simulink library "utils"  (R2007a)
settings: Solver=ode45  StartTime=0.0  StopTime=10.0  RelTol=1e-3
settings Model: Creator=aeagr  LastModifiedBy=aeagr

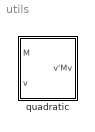
== system utils ==
  quadratic : Subsystem  mask(Quadratic){}

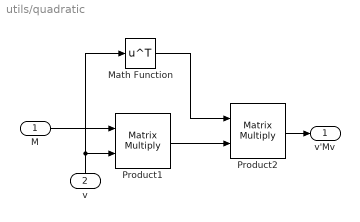
== system utils/quadratic ==
  M : Inport
  v : Inport  Port=2
  Math Function : Math  Operator=transpose  SaturateOnIntegerOverflow=on
  Product1 : Product  Multiplication=Matrix(*)  RndMeth=Zero
  Product2 : Product  Multiplication=Matrix(*)  RndMeth=Zero
  v'Mv : Outport
  wires:
  Product1/1 -> Product2/2
  Math Function/1 -> Product2/1
  v/1 -> Math Function/1, Product1/2
  M/1 -> Product1/1
  Product2/1 -> v'Mv/1
